simulink model "motore_caricorisonante"  (R2020b)
settings: Solver=ode45  StartTime=0.0  StopTime=10.0  RelTol=1e-3
values from neighbouring files (symbols this model uses):
  Beq = BeqEst    (= 1.0675e-06)    [PIDresonantdesign.m]
  den_B = [mld.Jb, Bb]    [PIDresonantdesign.m]
  Jeq = mot.J + mld.Jh/gbox.N^2    [PIDresonantdesign.m]
  k = mld.k    [PIDresonantdesign.m]
  tauSfEst = 0.0125    [PIDresonantdesign.m]
  Ts = 0.001    [PIDresonantdesign.m]
undefined symbols (not defined in the file or in its folder): daq, drv, gbox, mot, rads2rpm, sens
settings Model: Creator=giorgiadisaro  LastModifiedBy=giorgiadisaro

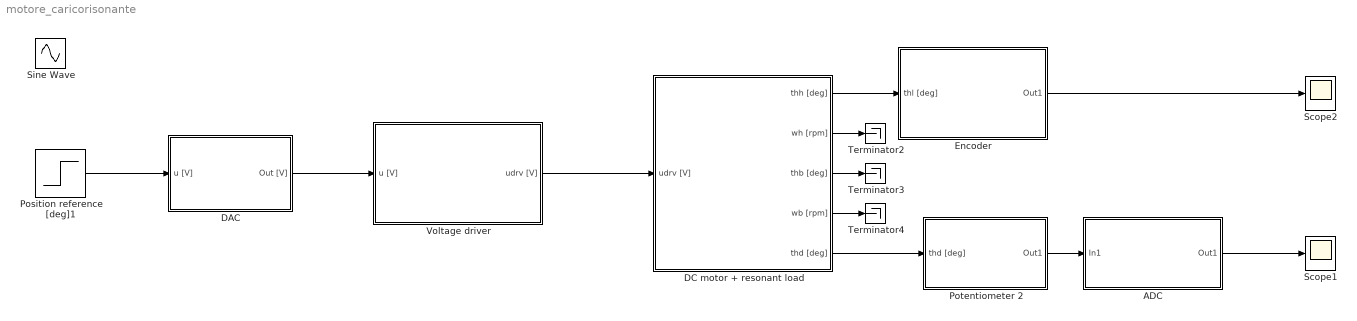
== system motore_caricorisonante ==
  ADC : Subsystem
  DAC : Subsystem
  DC motor + resonant load : Subsystem
  Encoder : Subsystem
  Position reference [deg]1 : Step  Time=0  After=50  SampleTime=0
  Potentiometer 2 : Subsystem
  Scope1 : Scope
  Scope2 : Scope
  Sine Wave : Sin  Amplitude=50  Frequency=120  SampleTime=0
  Terminator2 : Terminator
  Terminator3 : Terminator
  Terminator4 : Terminator
  Voltage driver : Subsystem
  wires:
  DAC/1(Out [V]) -> Voltage driver/1(u [V])
  Voltage driver/1(udrv [V]) -> DC motor + resonant load/1(udrv [V])
  Potentiometer 2/1(Out1) -> ADC/1(In1)
  DC motor + resonant load/5(thd [deg]) -> Potentiometer 2/1(thd [deg])
  ADC/1(Out1) -> Scope1/1
  DC motor + resonant load/2(wh [rpm]) -> Terminator2/1
  DC motor + resonant load/3(thb [deg]) -> Terminator3/1
  DC motor + resonant load/4(wb [rpm]) -> Terminator4/1
  DC motor + resonant load/1("thh [deg] ") -> Encoder/1("thl [deg] ")
  Encoder/1(Out1) -> Scope2/1
  Position reference [deg]1/1 -> DAC/1(u [V])

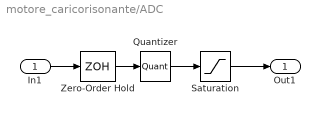
== system motore_caricorisonante/ADC ==
  In1 : Inport
  Quantizer : Quantizer  QuantizationInterval=daq.adc.q
  Saturation : Saturate  UpperLimit=daq.adc.fs  LowerLimit=-daq.adc.fs
  Zero-Order Hold : ZeroOrderHold  SampleTime=Ts
  Out1 : Outport
  wires:
  Saturation/1 -> Out1/1
  Quantizer/1 -> Saturation/1
  Zero-Order Hold/1 -> Quantizer/1
  In1/1 -> Zero-Order Hold/1

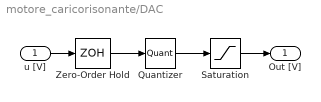
== system motore_caricorisonante/DAC ==
  u [V] : Inport
  Quantizer : Quantizer  QuantizationInterval=daq.dac.q
  Saturation : Saturate  UpperLimit=daq.dac.fs  LowerLimit=-daq.dac.fs
  Zero-Order Hold : ZeroOrderHold  SampleTime=Ts
  Out [V] : Outport
  wires:
  u [V]/1 -> Zero-Order Hold/1
  Zero-Order Hold/1 -> Quantizer/1
  Quantizer/1 -> Saturation/1
  Saturation/1 -> Out [V]/1

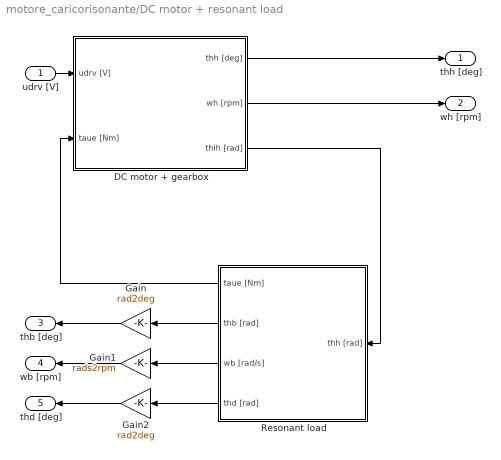
== system motore_caricorisonante/DC motor + resonant load ==
  udrv [V] : Inport
  DC motor + gearbox : Subsystem
  Gain : Gain  Gain=rad2deg
  Gain1 : Gain  Gain=rads2rpm
  Gain2 : Gain  Gain=rad2deg
  Resonant load : Subsystem
  "thh [deg] " : Outport
  wh [rpm] : Outport  Port=2
  thb [deg] : Outport  Port=3
  wb [rpm] : Outport  Port=4
  thd [deg] : Outport  Port=5
  wires:
  DC motor + gearbox/3(thlh [rad]) -> Resonant load/1(thh [rad])
  DC motor + gearbox/1("thh [deg] ") -> "thh [deg] "/1
  Resonant load/1(taue [Nm]) -> DC motor + gearbox/2(taue [Nm])
  udrv [V]/1 -> DC motor + gearbox/1(udrv [V])
  DC motor + gearbox/2(wh [rpm]) -> wh [rpm]/1
  Resonant load/2(thb [rad]) -> Gain/1
  Gain/1 -> thb [deg]/1
  Gain1/1 -> wb [rpm]/1
  Resonant load/3(wb [rad/s]) -> Gain1/1
  Resonant load/4(thd [rad]) -> Gain2/1
  Gain2/1 -> thd [deg]/1

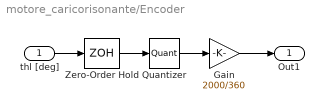
== system motore_caricorisonante/Encoder ==
  "thl [deg] " : Inport
  Gain : Gain  Gain=2000/360
  Quantizer : Quantizer  QuantizationInterval=360/(500*4)
  Zero-Order Hold : ZeroOrderHold  SampleTime=Ts
  Out1 : Outport
  wires:
  "thl [deg] "/1 -> Zero-Order Hold/1
  Zero-Order Hold/1 -> Quantizer/1
  Quantizer/1 -> Gain/1
  Gain/1 -> Out1/1

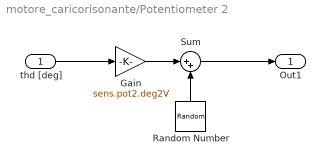
== system motore_caricorisonante/Potentiometer 2 ==
  thd [deg] : Inport
  Gain : Gain  Gain=sens.pot2.deg2V
  Random Number : RandomNumber  Variance=sens.pot2.noise.var  SampleTime=Ts
  Sum : Sum  Inputs=|++
  Out1 : Outport
  wires:
  thd [deg]/1 -> Gain/1
  Gain/1 -> Sum/1
  Sum/1 -> Out1/1
  Random Number/1 -> Sum/2

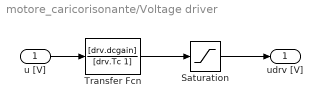
== system motore_caricorisonante/Voltage driver ==
  u [V] : Inport
  Saturation : Saturate  UpperLimit=drv.outmax  LowerLimit=-drv.outmax
  Transfer Fcn : TransferFcn  Numerator=[drv.dcgain]  Denominator=[drv.Tc 1]
  udrv [V] : Outport
  wires:
  u [V]/1 -> Transfer Fcn/1
  Transfer Fcn/1 -> Saturation/1
  Saturation/1 -> udrv [V]/1

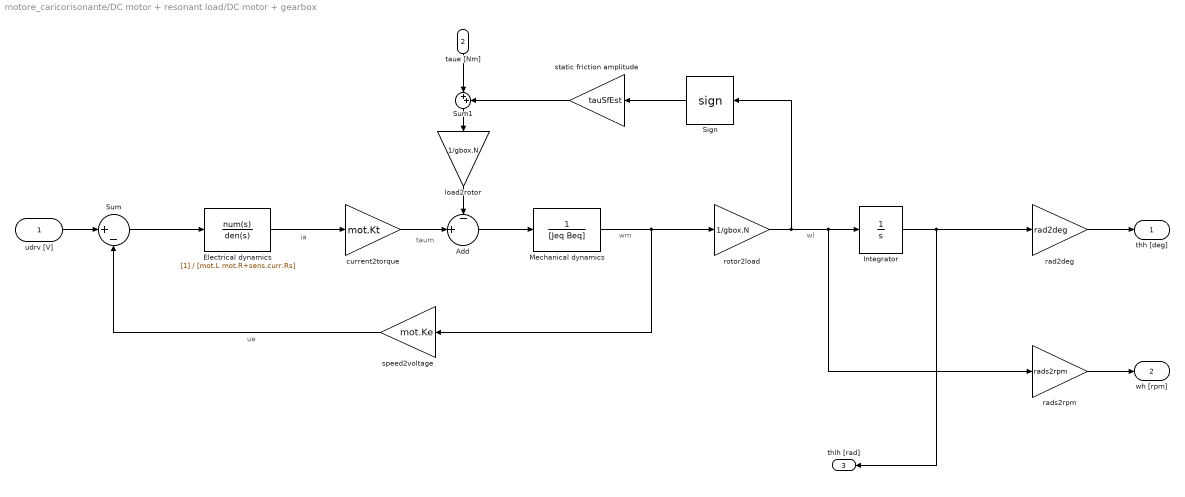
== system motore_caricorisonante/DC motor + resonant load/DC motor + gearbox ==
  note: wl
  note: wm
  note: ue
  note: taum
  note: ia
  udrv [V] : Inport
  taue [Nm] : Inport  Port=2
  Add : Sum  Inputs=-|+||
  Electrical dynamics : TransferFcn  Denominator=[mot.L mot.R+sens.curr.Rs]
  Integrator : Integrator
  Mechanical dynamics : TransferFcn  Denominator=[Jeq Beq]
  Sign : Signum  ZeroCross=off
  Sum : Sum  Inputs=|+-
  Sum1 : Sum  Inputs=|++
  current2torque : Gain  Gain=mot.Kt
  load2rotor : Gain  Gain=1/gbox.N
  rad2deg : Gain  Gain=rad2deg
  rads2rpm : Gain  Gain=rads2rpm
  rotor2load : Gain  Gain=1/gbox.N
  speed2voltage : Gain  Gain=mot.Ke
  static friction amplitude : Gain  Gain=tauSfEst
  "thh [deg] " : Outport
  wh [rpm] : Outport  Port=2
  thlh [rad] : Outport  Port=3
  wires:
  udrv [V]/1 -> Sum/1
  Electrical dynamics/1 -> current2torque/1
  current2torque/1 -> Add/2
  load2rotor/1 -> Add/1
  Sign/1 -> static friction amplitude/1
  speed2voltage/1 -> Sum/2
  rad2deg/1 -> "thh [deg] "/1
  Add/1 -> Mechanical dynamics/1
  Mechanical dynamics/1 -> speed2voltage/1, rotor2load/1
  rads2rpm/1 -> wh [rpm]/1
  Sum/1 -> Electrical dynamics/1
  rotor2load/1 -> Sign/1, rads2rpm/1, Integrator/1
  Integrator/1 -> thlh [rad]/1, rad2deg/1
  Sum1/1 -> load2rotor/1
  static friction amplitude/1 -> Sum1/2
  taue [Nm]/1 -> Sum1/1

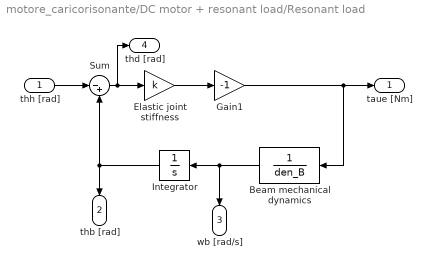
== system motore_caricorisonante/DC motor + resonant load/Resonant load ==
  thh [rad] : Inport
  Beam mechanical dynamics : TransferFcn  Denominator=den_B
  Elastic joint stiffness : Gain  Gain=k
  Gain1 : Gain  Gain=-1
  Integrator : Integrator
  Sum : Sum  Inputs=|-+
  taue [Nm] : Outport
  thb [rad] : Outport  Port=2
  wb [rad/s] : Outport  Port=3
  thd [rad] : Outport  Port=4
  wires:
  thh [rad]/1 -> Sum/1
  Integrator/1 -> thb [rad]/1, Sum/2
  Beam mechanical dynamics/1 -> Integrator/1, wb [rad/s]/1
  Sum/1 -> thd [rad]/1, Elastic joint stiffness/1
  Elastic joint stiffness/1 -> Gain1/1
  Gain1/1 -> Beam mechanical dynamics/1, taue [Nm]/1
